simulink model "abs2"  (R2015a)
settings: Solver=ode45  StartTime=0.0  StopTime=1  RelTol=1e-3
libraries: powerlib x26
settings Model: Creator=Yaman  LastModifiedBy=MBK

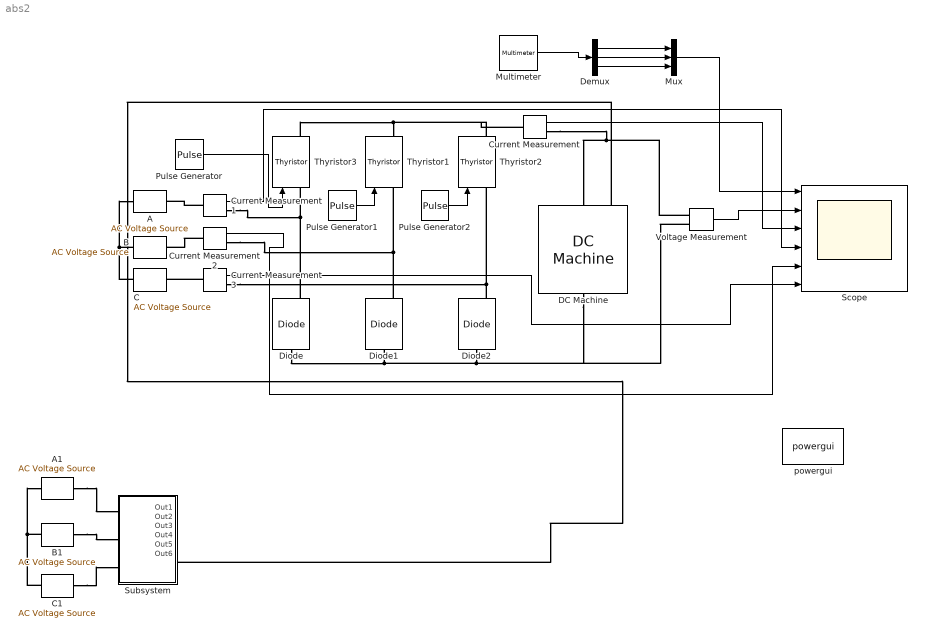
== system abs2 ==
  A : powerlib/Electrical Sources/AC Voltage Source  Amplitude=295  Phase=0  Frequency=50  SampleTime=0  Measurements=Voltage
  A1 : powerlib/Electrical Sources/AC Voltage Source  Amplitude=295  Phase=0  Frequency=50  SampleTime=0  Measurements=Voltage
  B : powerlib/Electrical Sources/AC Voltage Source  Amplitude=295  Phase=-120  Frequency=50  SampleTime=0  Measurements=Voltage
  B1 : powerlib/Electrical Sources/AC Voltage Source  Amplitude=295  Phase=-120  Frequency=50  SampleTime=0  Measurements=Voltage
  C : powerlib/Electrical Sources/AC Voltage Source  Amplitude=295  Phase=-240  Frequency=50  SampleTime=0  Measurements=Voltage
  C1 : powerlib/Electrical Sources/AC Voltage Source  Amplitude=295  Phase=-240  Frequency=50  SampleTime=0  Measurements=Voltage
  Current Measurement{,1..3} (4 alike) : powerlib/Measurements/Current Measurement  PhasorSimulation=off  OutputType=Complex  PSBequivalent=0
  DC Machine : powerlib/Machines/DC Machine  PresetModel=No  MechanicalLoad=Torque TL  FieldType=Wound  ShowDetailedParameters=on  MeasurementBus=off  RLa=[0.78 0.2]  RLf=[150 112.5]  Laf=1.234  MachineConstant=Torque constant (N.m/A)  Ke=1.8  Kt=1.8  J=0.05  Bm=0.01  Tf=0  w0=1  Ifinit=1  TsPowergui=0  TsBlock=-1
  Demux : Demux  Outputs=3
  Diode : powerlib/Power Electronics/Diode  Ron=0.001  Lon=0  Vf=0.8  IC=0  UseSnubber=off  Rs=500  Cs=250e-9  Measurements=on
  Diode1 : powerlib/Power Electronics/Diode  Ron=0.001  Lon=0  Vf=0.8  IC=0  UseSnubber=off  Rs=500  Cs=250e-9  Measurements=on
  Diode2 : powerlib/Power Electronics/Diode  Ron=0.001  Lon=0  Vf=0.8  IC=0  UseSnubber=off  Rs=500  Cs=250e-9  Measurements=on
  Multimeter : powerlib/Measurements/Multimeter  PhasorSimulation=off  OutputType=Complex  sel=[6 4 2]  L=6  Gain=[1 1 1]  yselected={'Usrc: A','Usrc: B','Usrc: C'};  PSBOutputType=1  PSBequivalent=0  AxesSetting=[0,0.1,-100,100]  Display=0  SavedBlockNames=-11
  Mux : Mux  Inputs=3
  Pulse Generator : DiscretePulseGenerator  PulseType=Time based  Amplitude=5  Period=0.02  PulseWidth=33.3333  PhaseDelay=(30+60)*0.02/360
  Pulse Generator1 : DiscretePulseGenerator  PulseType=Time based  Amplitude=5  Period=0.02  PulseWidth=33.333  PhaseDelay=(150+60)*0.02/360
  Pulse Generator2 : DiscretePulseGenerator  PulseType=Time based  Amplitude=5  Period=0.02  PulseWidth=33.333  PhaseDelay=(270+60)*0.02/360
  Scope : Scope  NumInputPorts=6
      settings: YMin=-100~-100~-750~-750~-750~-5  YMax=600~700~750~750~750~5
  Subsystem : Subsystem
  Thyristor1 : powerlib/Power Electronics/Thyristor  Ron=0.001  Lon=0  Vf=0.8  IC=0  Rs=500  Cs=250e-9  Measurements=on
  Thyristor2 : powerlib/Power Electronics/Thyristor  Ron=0.001  Lon=0  Vf=0.8  IC=0  Rs=500  Cs=250e-9  Measurements=on
  Thyristor3 : powerlib/Power Electronics/Thyristor  Ron=0.001  Lon=0  Vf=0.8  IC=0  Rs=500  Cs=250e-9  Measurements=on
  Voltage Measurement : powerlib/Measurements/Voltage Measurement  PhasorSimulation=off  OutputType=Complex  PSBequivalent=0
  powergui : powerlib/powergui  Priority=1  SimulationMode=Continuous  SolverType=Tustin/Backward Euler (TBE)  SampleTime=50e-6  frequency=60  SPID=off  DisableSnubberDevices=off  DisableRonSwitches=off  DisableVfSwitches=off  SwTol=0  DisplayEquations=off  Interpol=off  methode=off  Ts=100  FunctionMessages=off  echomessages=off  HookPort=off  EnableUseOfTLC=off  x0status=blocks  frequencyindice=50  Pbase=100e6  ErrMax=1e-4  Iterations=50  UnitsV=kV  UnitsW=MW  buscounter=0  RestoreLinks=warning  ResistiveCurrentMeasurement=off  Frange=[0:2:500]  Ylog=off  Xlog=on  ShowGrid=off  save=off  variable=ZData  structure=0  ZoomFFT=off  StartTime=0.0  cycles=1  DisplayStyle=1  fundamental=60  FreqAxis=off  MaxFrequency=1000  frequencyindicesteady=1  RmsSteady=1  display=off
  wires:
  Pulse Generator/1 -> Thyristor3/1
  Pulse Generator1/1 -> Thyristor1/1
  Pulse Generator2/1 -> Thyristor2/1
  Voltage Measurement/1 -> Scope/2
  Current Measurement/1 -> Scope/3
  Current Measurement1/1 -> Scope/4
  Current Measurement2/1 -> Scope/5
  Current Measurement3/1 -> Scope/6
  Multimeter/1 -> Demux/1
  Demux/1 -> Mux/1
  Demux/2 -> Mux/2
  Demux/3 -> Mux/3
  Mux/1 -> Scope/1
  connections:
  Diode/LConn1 -- DC Machine/RConn1 -- Voltage Measurement/LConn2 -- Diode2/LConn1 -- Diode1/LConn1
  B1/LConn1 -- C1/LConn1 -- A1/LConn1
  B1/RConn1 -- Subsystem/LConn2
  A1/RConn1 -- Subsystem/LConn1
  C1/RConn1 -- Subsystem/LConn3
  DC Machine/LConn2 -- Subsystem/RConn1
  Diode1/RConn1 -- Current Measurement2/RConn1 -- Thyristor1/LConn1
  Diode2/RConn1 -- Current Measurement3/RConn1 -- Thyristor2/LConn1
  Diode/RConn1 -- Current Measurement1/RConn1 -- Thyristor3/LConn1
  Thyristor3/RConn1 -- Current Measurement/LConn1 -- Thyristor2/RConn1 -- Thyristor1/RConn1
  Voltage Measurement/LConn1 -- DC Machine/LConn1 -- Current Measurement/RConn1
  Current Measurement1/LConn1 -- A/RConn1
  Current Measurement2/LConn1 -- B/RConn1
  Current Measurement3/LConn1 -- C/RConn1
  B/LConn1 -- C/LConn1 -- A/LConn1

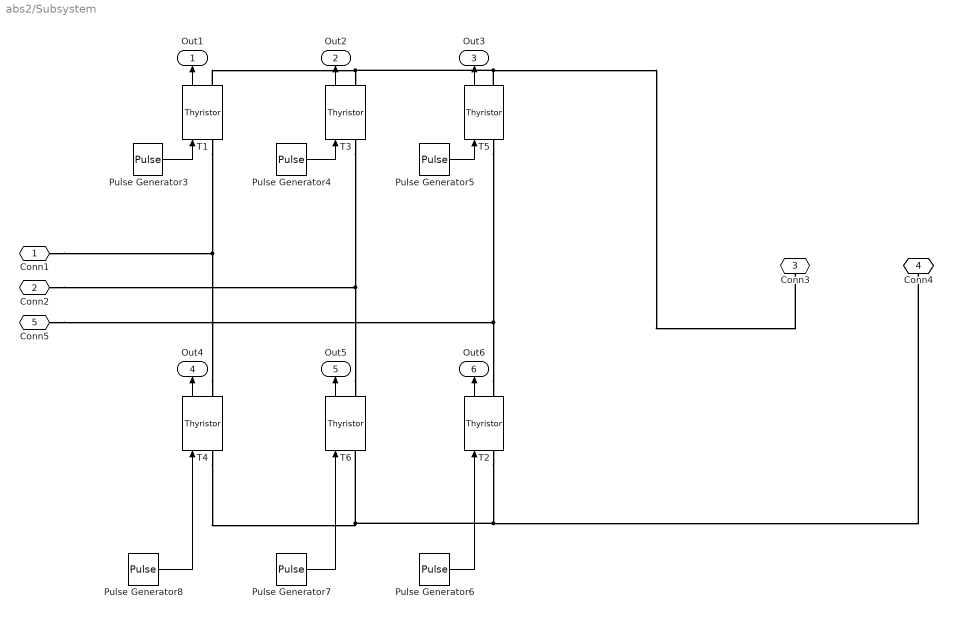
== system abs2/Subsystem ==
  Pulse Generator3 : DiscretePulseGenerator  PulseType=Time based  Period=0.02  PulseWidth=33.333  PhaseDelay=30*0.02/360
  Pulse Generator4 : DiscretePulseGenerator  PulseType=Time based  Period=0.02  PulseWidth=33.333  PhaseDelay=150*0.02/360
  Pulse Generator5 : DiscretePulseGenerator  PulseType=Time based  Period=0.02  PulseWidth=33.333  PhaseDelay=270*0.02/360
  Pulse Generator6 : DiscretePulseGenerator  PulseType=Time based  Period=0.02  PulseWidth=33.333  PhaseDelay=90*0.02/360
  Pulse Generator7 : DiscretePulseGenerator  PulseType=Time based  Period=0.02  PulseWidth=33.333  PhaseDelay=330*0.02/360
  Pulse Generator8 : DiscretePulseGenerator  PulseType=Time based  Period=0.02  PulseWidth=33.333  PhaseDelay=210*0.02/360
  T{1..6} (6 alike) : powerlib/Power Electronics/Thyristor  Ron=0.001  Lon=0  Vf=0.8  IC=0  Rs=500  Cs=250e-9  Measurements=on
  Conn1 : PMIOPort  Port=1  Side=Left
  Conn2 : PMIOPort  Port=2  Side=Left
  Conn3 : PMIOPort  Port=3  Side=Right
  Conn4 : PMIOPort  Port=4  Side=Right
  Conn5 : PMIOPort  Port=5  Side=Left
  Out1 : Outport
  Out2 : Outport  Port=2
  Out3 : Outport  Port=3
  Out4 : Outport  Port=4
  Out5 : Outport  Port=5
  Out6 : Outport  Port=6
  wires:
  T5/1 -> Out3/1
  T1/1 -> Out1/1
  T6/1 -> Out5/1
  T3/1 -> Out2/1
  T2/1 -> Out6/1
  T4/1 -> Out4/1
  Pulse Generator8/1 -> T4/1
  Pulse Generator3/1 -> T1/1
  Pulse Generator5/1 -> T5/1
  Pulse Generator4/1 -> T3/1
  Pulse Generator6/1 -> T2/1
  Pulse Generator7/1 -> T6/1
  connections:
  T4/RConn1 -- T1/LConn1 -- Conn1/RConn1
  T6/RConn1 -- T3/LConn1 -- Conn2/RConn1
  T2/RConn1 -- T5/LConn1 -- Conn5/RConn1
  T3/RConn1 -- T1/RConn1 -- T5/RConn1 -- Conn3/RConn1
  T2/LConn1 -- T6/LConn1 -- T4/LConn1 -- Conn4/RConn1
